simulink model "gap_generation_platoon"  (R2019a)
settings: Solver=VariableStepAuto  StartTime=0.0  StopTime=50  RelTol=1e-3
libraries: simulink x68, powerlib_meascontrol x7, autolibshared x7
(part 3 of 3)

== system gap_generation_platoon/p2/ACC ==
  note: If there's no leader or the leader
      | is too far away, use velocity control
  note: Velocity control
  note: Switch logic (veh foll to vel control)
  note: Vehicle following
  currentStates : Inport
  leaderStates : Inport  Port=2
  lcFlag : Inport  Port=3
  ACC outputs : Scope  NumInputPorts=3
  AND : Logic  IconShape=distinctive  AllPortsSameDT=off  OutDataTypeStr=boolean
  AND1 : Logic  IconShape=distinctive  AllPortsSameDT=off  OutDataTypeStr=boolean
  Anti-windup gain : Gain  Gain=sqrt(Ki/Kd)
  Bus Selector : BusSelector  OutputSignals=X,Xdot,u
  Bus Selector1 : BusSelector  OutputSignals=X,Xdot
  Compare To Constant : simulink/Logic and Bit Operations/Compare To Constant  relop=<  const=2*maxHeadwayError  OutDataTypeStr=boolean
  Compare To Constant1 : simulink/Logic and Bit Operations/Compare To Constant  relop=>  const=0  OutDataTypeStr=boolean
  Gain3 : Gain  Gain=velFilterGain
  Headway error : Subsystem
  Integrator : Integrator  ExternalReset=either
  Integrator1 : Integrator  InitialCondition=vx0
  Integrator2 : Integrator
  Kd : Gain  Gain=Kd
  Ki : Gain  Gain=Ki
  Kp : Gain  Gain=Kp
  Mux : Mux  Inputs=2
  NOT : Logic  Operator=NOT  IconShape=distinctive  AllPortsSameDT=off  OutDataTypeStr=boolean
  Rate Limiter : RateLimiter  RisingSlewLimit=maxJerk  FallingSlewLimit=minJerk  SampleTimeMode=inherited
  Saturation : Saturate  UpperLimit=maxAcceleration  LowerLimit=minAcceleration
  Saturation1 : Saturate  UpperLimit=maxHeadwayError  LowerLimit=minHeadwayError
  Scope : Scope  NumInputPorts=3
  Sum : Sum  Inputs=-+|
  Sum1 : Sum  Inputs=+++
  Sum2 : Sum  Inputs=|+-
  Sum3 : Sum
  Sum4 : Sum  Inputs=+-
  Sum5 : Sum  Inputs=-+|
  Switch : Switch  Criteria=u2 > Threshold
  Switch1 : Switch  Criteria=u2 > Threshold
  comf saturation : Saturate  UpperLimit=maxAcceleration/2  LowerLimit=minAcceleration/4
  safe saturation : Saturate  UpperLimit=maxAcceleration  LowerLimit=minAcceleration
  velKi : Gain  Gain=velKi
  velKp : Gain  Gain=velKp
  u : Outport
  errors : Outport  Port=2
  gap : Outport  Port=3
  wires:
  comf saturation/1 -> Switch1/1
  safe saturation/1 -> Switch1/3
  Switch1/1 -> Rate Limiter/1
  AND1/1 -> Switch1/2
  [lcFlag] -> AND1/2
  NOT/1 -> AND1/1
  [unsafeFlag] -> NOT/1
  Headway error/3(unsafeFlag) -> [unsafeFlag]
  [realInput] -> Sum4/2
  Bus Selector/3 -> [realInput]  "<u>"
  Bus Selector1/1 -> Headway error/3(xl), Compare To Constant1/1  "<X>"
  leaderStates/1 -> Bus Selector1/1
  Bus Selector/1 -> Headway error/1(xf)  "<X>"
  currentStates/1 -> Bus Selector/1
  lcFlag/1 -> Headway error/4(lcFlag), [lcFlag]
  Compare To Constant1/1 -> AND/1
  Compare To Constant/1 -> AND/2
  AND/1 -> ACC outputs/2, Switch/2, Integrator/2
  Anti-windup gain/1 -> Sum5/1
  Integrator/1 -> Scope/1, Sum1/1
  Ki/1 -> Sum5/2
  velKp/1 -> Sum3/1
  Rate Limiter/1 -> u/1  "sat(u)"
  Sum5/1 -> Integrator/1
  Sum4/1 -> Anti-windup gain/1
  Mux/1 -> errors/1
  Sum/1 -> Integrator2/1, velKp/1, Kd/1, Mux/2
  Sum3/1 -> Switch/3, ACC outputs/3
  Sum1/1 -> ACC outputs/1, Switch/1
  Switch/1 -> comf saturation/1, safe saturation/1, Sum4/1  "u"
  velKi/1 -> Sum3/2
  Integrator2/1 -> velKi/1
  Headway error/2("gap ") -> gap/1
  Saturation1/1 -> Ki/1, Kp/1
  Sum2/1 -> Gain3/1
  Bus Selector1/2 -> Sum2/1  "<Xdot>"
  Integrator1/1 -> Sum/2, Sum2/2
  Saturation/1 -> Integrator1/1
  Gain3/1 -> Saturation/1
  Kp/1 -> Sum1/2, Scope/2
  Kd/1 -> Sum1/3, Scope/3
  Bus Selector/2 -> Sum/1, Headway error/2(vf)  "<Xdot>"
  Headway error/1(eh) -> Compare To Constant/1, Mux/1, Saturation1/1

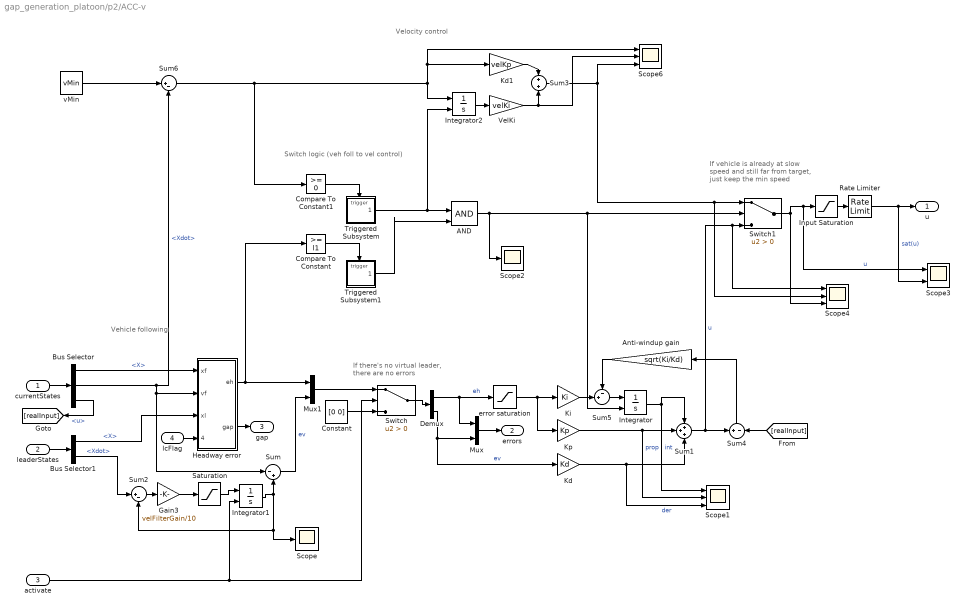
== system gap_generation_platoon/p2/ACC-v ==
  note: If there's no virtual leader,
      | there are no errors
  note: If vehicle is already at slow
      | speed and still far from target,
      | just keep the min speed
  note: Velocity control
  note: Switch logic (veh foll to vel control)
  note: Vehicle following
  currentStates : Inport
  leaderStates : Inport  Port=2
  activate : Inport  Port=3
  lcFlag : Inport  Port=4
  AND : Logic  IconShape=distinctive  AllPortsSameDT=off  OutDataTypeStr=boolean
  Anti-windup gain : Gain  Gain=sqrt(Ki/Kd)
  Bus Selector : BusSelector  OutputSignals=X,Xdot,u
  Bus Selector1 : BusSelector  OutputSignals=X,Xdot
  Compare To Constant : simulink/Logic and Bit Operations/Compare To Constant  relop=>=  const=l1  OutDataTypeStr=boolean
  Compare To Constant1 : simulink/Logic and Bit Operations/Compare To Constant  relop=>=  const=0  OutDataTypeStr=boolean
  Constant : Constant  Value=[0 0]
  Demux : Demux  Outputs=2
  Gain3 : Gain  Gain=velFilterGain/10
  Headway error : Subsystem
  Input Saturation : Saturate  UpperLimit=maxAcceleration/2  LowerLimit=minAcceleration/4
  Integrator : Integrator  ExternalReset=falling
  Integrator1 : Integrator  ExternalReset=rising  InitialCondition=vx0
  Integrator2 : Integrator  ExternalReset=rising
  Kd : Gain  Gain=Kd
  Kd1 : Gain  Gain=velKp
  Ki : Gain  Gain=Ki
  Kp : Gain  Gain=Kp
  Mux : Mux  Inputs=2
  Mux1 : Mux  Inputs=2
  Rate Limiter : RateLimiter  RisingSlewLimit=maxJerk/2  FallingSlewLimit=minJerk/3  SampleTimeMode=inherited
  Saturation : Saturate  UpperLimit=maxAcceleration  LowerLimit=minAcceleration
  Scope : Scope
  Scope1 : Scope  NumInputPorts=3
  Scope2 : Scope
  Scope3 : Scope  NumInputPorts=2
  Scope4 : Scope  NumInputPorts=3
  Scope6 : Scope  NumInputPorts=3
  Sum : Sum  Inputs=|-+
  Sum1 : Sum  Inputs=+++
  Sum2 : Sum  Inputs=|+-
  Sum3 : Sum
  Sum4 : Sum  Inputs=+-
  Sum5 : Sum  Inputs=-+|
  Sum6 : Sum  Inputs=|+-
  Switch : Switch  Criteria=u2 > Threshold
  Switch1 : Switch  Criteria=u2 > Threshold
  Triggered Subsystem : Subsystem  TreatAsAtomicUnit=on
  Triggered Subsystem1 : Subsystem  TreatAsAtomicUnit=on
  VelKi : Gain  Gain=velKi
  error saturation : Saturate  UpperLimit=maxHeadwayError  LowerLimit=minHeadwayError/10
  vMin : Constant  Value=vMin
  u : Outport
  errors : Outport  Port=2
  gap : Outport  Port=3
  wires:
  AND/1 -> Scope2/1, Integrator/2, Switch1/2
  Triggered Subsystem1/1(Out1) -> AND/2
  lcFlag/1 -> Headway error/4(lcFlag)
  Bus Selector/3 -> [realInput]  "<u>"
  Bus Selector1/1 -> Headway error/3(xl)  "<X>"
  leaderStates/1 -> Bus Selector1/1
  Bus Selector/2 -> Sum/1, Headway error/2(vf), Sum6/2  "<Xdot>"
  Bus Selector/1 -> Headway error/1(xf)  "<X>"
  currentStates/1 -> Bus Selector/1
  [realInput] -> Sum4/2
  Triggered Subsystem/1(Out1) -> Integrator2/2, AND/1
  Sum5/1 -> Integrator/1
  error saturation/1 -> Ki/1, Kp/1
  Switch1/1 -> Scope4/3, Input Saturation/1, Scope3/1  "u"
  vMin/1 -> Sum6/1
  VelKi/1 -> Sum3/2, Scope6/2
  Kd1/1 -> Sum3/1
  Integrator2/1 -> VelKi/1
  Sum3/1 -> Switch1/1, Scope4/2, Scope6/3
  Sum6/1 -> Compare To Constant1/1, Integrator2/1, Kd1/1, Scope6/1
  Compare To Constant/1 -> Triggered Subsystem1/Trigger
  Compare To Constant1/1 -> Triggered Subsystem/Trigger
  Rate Limiter/1 -> u/1, Scope3/2  "sat(u)"
  Constant/1 -> Switch/3
  activate/1 -> Integrator1/2, Switch/2
  Mux1/1 -> Switch/1
  Switch/1 -> Demux/1
  Demux/2 -> Kd/1, Mux/2  "ev"
  Anti-windup gain/1 -> Sum5/1
  Ki/1 -> Sum5/2
  Sum4/1 -> Anti-windup gain/1
  Integrator/1 -> Scope1/1, Sum1/1  "int"
  Input Saturation/1 -> Rate Limiter/1
  Mux/1 -> errors/1
  Sum/1 -> Mux1/2  "ev"
  Sum1/1 -> Sum4/1, Switch1/3, Scope4/1  "u"
  Headway error/2("gap ") -> gap/1
  Demux/1 -> Mux/1, error saturation/1  "eh"
  Sum2/1 -> Gain3/1
  Bus Selector1/2 -> Sum2/1  "<Xdot>"
  Integrator1/1 -> Sum/2, Sum2/2, Scope/1
  Saturation/1 -> Integrator1/1
  Gain3/1 -> Saturation/1
  Kp/1 -> Sum1/2, Scope1/2  "prop"
  Kd/1 -> Sum1/3, Scope1/3  "der"
  Headway error/1(eh) -> Compare To Constant/1, Mux1/1

== system gap_generation_platoon/p2/Detect steady state ==
  errors : Inport
  virtual errors : Inport  Port=2
  ACC-v active : Inport  Port=3
  AND1 : Logic  IconShape=distinctive  AllPortsSameDT=off  OutDataTypeStr=boolean
  AND2 : Logic  IconShape=distinctive  AllPortsSameDT=off  OutDataTypeStr=boolean
  AND5 : Logic  IconShape=distinctive  AllPortsSameDT=off  OutDataTypeStr=boolean
  Abs : Abs
  Abs1 : Abs  ZeroCross=off
  Abs2 : Abs
  Abs3 : Abs  ZeroCross=off
  Compare To Constant{,1..3} (4 alike) : simulink/Logic and Bit Operations/Compare To Constant  relop=<=  const=0.5  OutDataTypeStr=boolean
  Demux : Demux  Outputs=2
  OR : Logic  Operator=OR  IconShape=distinctive  AllPortsSameDT=off  OutDataTypeStr=boolean
  Subsystem : Subsystem
  Transport Delay : TransportDelay
  Transport Delay1 : TransportDelay
  Out1 : Outport
  wires:
  ACC-v active/1 -> Subsystem/Enable
  Subsystem/1(Out1) -> OR/2
  virtual errors/1 -> Subsystem/1(virtual errors)
  AND5/1 -> OR/1
  OR/1 -> Out1/1
  AND2/1 -> AND5/2
  AND1/1 -> AND5/1
  Compare To Constant2/1 -> AND2/2
  Compare To Constant3/1 -> AND2/1
  Compare To Constant/1 -> AND1/2
  Compare To Constant1/1 -> AND1/1
  Demux/2 -> Transport Delay1/1, Abs3/1
  Demux/1 -> Transport Delay/1, Abs1/1
  Abs2/1 -> Compare To Constant2/1
  Transport Delay1/1 -> Abs2/1
  Abs3/1 -> Compare To Constant3/1
  errors/1 -> Demux/1
  Abs1/1 -> Compare To Constant1/1
  Transport Delay/1 -> Abs/1
  Abs/1 -> Compare To Constant/1

== system gap_generation_platoon/p2/Triggered Subsystem ==
  In1 : Inport
  Trigger : TriggerPort  VariantControl=Variant
  Out1 : Outport
  wires:
  In1/1 -> Out1/1

== system gap_generation_platoon/p3/ACC ==
  note: Vehicle following
  note: Switch logic (veh foll to vel control)
  note: Velocity control
  note: If there's no leader or the leader
      | is too far away, use velocity control
  currentStates : Inport
  leaderStates : Inport  Port=2
  lcFlag : Inport  Port=3
  ACC outputs : Scope  NumInputPorts=3
  AND : Logic  IconShape=distinctive  AllPortsSameDT=off  OutDataTypeStr=boolean
  AND1 : Logic  IconShape=distinctive  AllPortsSameDT=off  OutDataTypeStr=boolean
  Anti-windup gain : Gain  Gain=sqrt(Ki/Kd)
  Bus Selector : BusSelector  OutputSignals=X,Xdot,u
  Bus Selector1 : BusSelector  OutputSignals=X,Xdot
  Compare To Constant : simulink/Logic and Bit Operations/Compare To Constant  relop=<  const=2*maxHeadwayError  OutDataTypeStr=boolean
  Compare To Constant1 : simulink/Logic and Bit Operations/Compare To Constant  relop=>  const=0  OutDataTypeStr=boolean
  Gain3 : Gain  Gain=velFilterGain
  Headway error : Subsystem
  Integrator : Integrator  ExternalReset=either
  Integrator1 : Integrator  InitialCondition=vx0
  Integrator2 : Integrator
  Kd : Gain  Gain=Kd
  Ki : Gain  Gain=Ki
  Kp : Gain  Gain=Kp
  Mux : Mux  Inputs=2
  NOT : Logic  Operator=NOT  IconShape=distinctive  AllPortsSameDT=off  OutDataTypeStr=boolean
  Rate Limiter : RateLimiter  RisingSlewLimit=maxJerk  FallingSlewLimit=minJerk  SampleTimeMode=inherited
  Saturation : Saturate  UpperLimit=maxAcceleration  LowerLimit=minAcceleration
  Saturation1 : Saturate  UpperLimit=maxHeadwayError  LowerLimit=minHeadwayError
  Scope : Scope  NumInputPorts=3
  Sum : Sum  Inputs=-+|
  Sum1 : Sum  Inputs=+++
  Sum2 : Sum  Inputs=|+-
  Sum3 : Sum
  Sum4 : Sum  Inputs=+-
  Sum5 : Sum  Inputs=-+|
  Switch : Switch  Criteria=u2 > Threshold
  Switch1 : Switch  Criteria=u2 > Threshold
  comf saturation : Saturate  UpperLimit=maxAcceleration/2  LowerLimit=minAcceleration/4
  safe saturation : Saturate  UpperLimit=maxAcceleration  LowerLimit=minAcceleration
  velKi : Gain  Gain=velKi
  velKp : Gain  Gain=velKp
  u : Outport
  errors : Outport  Port=2
  gap : Outport  Port=3
  wires:
  Headway error/1(eh) -> Saturation1/1, Mux/1, Compare To Constant/1
  Bus Selector/2 -> Headway error/2(vf), Sum/1  "<Xdot>"
  Kd/1 -> Scope/3, Sum1/3
  Kp/1 -> Scope/2, Sum1/2
  Gain3/1 -> Saturation/1
  Saturation/1 -> Integrator1/1
  Integrator1/1 -> Sum2/2, Sum/2
  Bus Selector1/2 -> Sum2/1  "<Xdot>"
  Sum2/1 -> Gain3/1
  Saturation1/1 -> Kp/1, Ki/1
  Headway error/2("gap ") -> gap/1
  Integrator2/1 -> velKi/1
  velKi/1 -> Sum3/2
  Switch/1 -> Sum4/1, safe saturation/1, comf saturation/1  "u"
  Sum1/1 -> Switch/1, ACC outputs/1
  Sum3/1 -> ACC outputs/3, Switch/3
  Sum/1 -> Mux/2, Kd/1, velKp/1, Integrator2/1
  Mux/1 -> errors/1
  Sum4/1 -> Anti-windup gain/1
  Sum5/1 -> Integrator/1
  Rate Limiter/1 -> u/1  "sat(u)"
  velKp/1 -> Sum3/1
  Ki/1 -> Sum5/2
  Integrator/1 -> Sum1/1, Scope/1
  Anti-windup gain/1 -> Sum5/1
  AND/1 -> Integrator/2, Switch/2, ACC outputs/2
  Compare To Constant/1 -> AND/2
  Compare To Constant1/1 -> AND/1
  lcFlag/1 -> [lcFlag], Headway error/4(lcFlag)
  currentStates/1 -> Bus Selector/1
  Bus Selector/1 -> Headway error/1(xf)  "<X>"
  leaderStates/1 -> Bus Selector1/1
  Bus Selector1/1 -> Compare To Constant1/1, Headway error/3(xl)  "<X>"
  Bus Selector/3 -> [realInput]  "<u>"
  [realInput] -> Sum4/2
  Headway error/3(unsafeFlag) -> [unsafeFlag]
  [unsafeFlag] -> NOT/1
  NOT/1 -> AND1/1
  [lcFlag] -> AND1/2
  AND1/1 -> Switch1/2
  Switch1/1 -> Rate Limiter/1
  safe saturation/1 -> Switch1/3
  comf saturation/1 -> Switch1/1

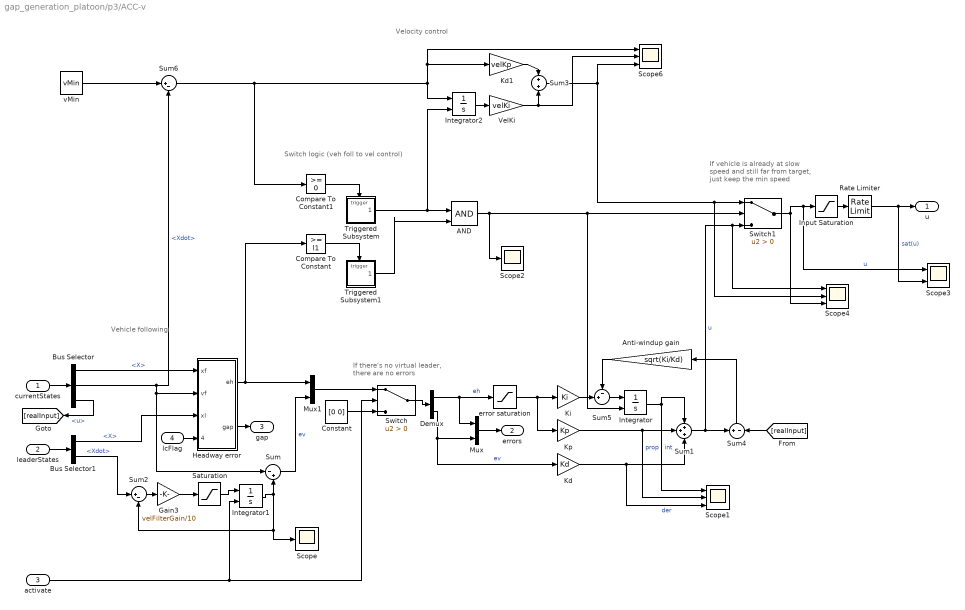
== system gap_generation_platoon/p3/ACC-v ==
  note: Vehicle following
  note: Switch logic (veh foll to vel control)
  note: Velocity control
  note: If vehicle is already at slow
      | speed and still far from target,
      | just keep the min speed
  note: If there's no virtual leader,
      | there are no errors
  currentStates : Inport
  leaderStates : Inport  Port=2
  activate : Inport  Port=3
  lcFlag : Inport  Port=4
  AND : Logic  IconShape=distinctive  AllPortsSameDT=off  OutDataTypeStr=boolean
  Anti-windup gain : Gain  Gain=sqrt(Ki/Kd)
  Bus Selector : BusSelector  OutputSignals=X,Xdot,u
  Bus Selector1 : BusSelector  OutputSignals=X,Xdot
  Compare To Constant : simulink/Logic and Bit Operations/Compare To Constant  relop=>=  const=l1  OutDataTypeStr=boolean
  Compare To Constant1 : simulink/Logic and Bit Operations/Compare To Constant  relop=>=  const=0  OutDataTypeStr=boolean
  Constant : Constant  Value=[0 0]
  Demux : Demux  Outputs=2
  Gain3 : Gain  Gain=velFilterGain/10
  Headway error : Subsystem
  Input Saturation : Saturate  UpperLimit=maxAcceleration/2  LowerLimit=minAcceleration/4
  Integrator : Integrator  ExternalReset=falling
  Integrator1 : Integrator  ExternalReset=rising  InitialCondition=vx0
  Integrator2 : Integrator  ExternalReset=rising
  Kd : Gain  Gain=Kd
  Kd1 : Gain  Gain=velKp
  Ki : Gain  Gain=Ki
  Kp : Gain  Gain=Kp
  Mux : Mux  Inputs=2
  Mux1 : Mux  Inputs=2
  Rate Limiter : RateLimiter  RisingSlewLimit=maxJerk/2  FallingSlewLimit=minJerk/3  SampleTimeMode=inherited
  Saturation : Saturate  UpperLimit=maxAcceleration  LowerLimit=minAcceleration
  Scope : Scope
  Scope1 : Scope  NumInputPorts=3
  Scope2 : Scope
  Scope3 : Scope  NumInputPorts=2
  Scope4 : Scope  NumInputPorts=3
  Scope6 : Scope  NumInputPorts=3
  Sum : Sum  Inputs=|-+
  Sum1 : Sum  Inputs=+++
  Sum2 : Sum  Inputs=|+-
  Sum3 : Sum
  Sum4 : Sum  Inputs=+-
  Sum5 : Sum  Inputs=-+|
  Sum6 : Sum  Inputs=|+-
  Switch : Switch  Criteria=u2 > Threshold
  Switch1 : Switch  Criteria=u2 > Threshold
  Triggered Subsystem : Subsystem  TreatAsAtomicUnit=on
  Triggered Subsystem1 : Subsystem  TreatAsAtomicUnit=on
  VelKi : Gain  Gain=velKi
  error saturation : Saturate  UpperLimit=maxHeadwayError  LowerLimit=minHeadwayError/10
  vMin : Constant  Value=vMin
  u : Outport
  errors : Outport  Port=2
  gap : Outport  Port=3
  wires:
  Headway error/1(eh) -> Mux1/1, Compare To Constant/1
  Kd/1 -> Scope1/3, Sum1/3  "der"
  Kp/1 -> Scope1/2, Sum1/2  "prop"
  Gain3/1 -> Saturation/1
  Saturation/1 -> Integrator1/1
  Integrator1/1 -> Scope/1, Sum2/2, Sum/2
  Bus Selector1/2 -> Sum2/1  "<Xdot>"
  Sum2/1 -> Gain3/1
  Demux/1 -> error saturation/1, Mux/1  "eh"
  Headway error/2("gap ") -> gap/1
  Sum1/1 -> Scope4/1, Switch1/3, Sum4/1  "u"
  Sum/1 -> Mux1/2  "ev"
  Mux/1 -> errors/1
  Input Saturation/1 -> Rate Limiter/1
  Integrator/1 -> Sum1/1, Scope1/1  "int"
  Sum4/1 -> Anti-windup gain/1
  Ki/1 -> Sum5/2
  Anti-windup gain/1 -> Sum5/1
  Demux/2 -> Mux/2, Kd/1  "ev"
  Switch/1 -> Demux/1
  Mux1/1 -> Switch/1
  activate/1 -> Switch/2, Integrator1/2
  Constant/1 -> Switch/3
  Rate Limiter/1 -> Scope3/2, u/1  "sat(u)"
  Compare To Constant1/1 -> Triggered Subsystem/Trigger
  Compare To Constant/1 -> Triggered Subsystem1/Trigger
  Sum6/1 -> Scope6/1, Kd1/1, Integrator2/1, Compare To Constant1/1
  Sum3/1 -> Scope6/3, Scope4/2, Switch1/1
  Integrator2/1 -> VelKi/1
  Kd1/1 -> Sum3/1
  VelKi/1 -> Scope6/2, Sum3/2
  vMin/1 -> Sum6/1
  Switch1/1 -> Scope3/1, Input Saturation/1, Scope4/3  "u"
  error saturation/1 -> Kp/1, Ki/1
  Sum5/1 -> Integrator/1
  Triggered Subsystem/1(Out1) -> AND/1, Integrator2/2
  [realInput] -> Sum4/2
  currentStates/1 -> Bus Selector/1
  Bus Selector/1 -> Headway error/1(xf)  "<X>"
  Bus Selector/2 -> Sum6/2, Headway error/2(vf), Sum/1  "<Xdot>"
  leaderStates/1 -> Bus Selector1/1
  Bus Selector1/1 -> Headway error/3(xl)  "<X>"
  Bus Selector/3 -> [realInput]  "<u>"
  lcFlag/1 -> Headway error/4(lcFlag)
  Triggered Subsystem1/1(Out1) -> AND/2
  AND/1 -> Switch1/2, Integrator/2, Scope2/1

== system gap_generation_platoon/p3/Detect steady state ==
  errors : Inport
  virtual errors : Inport  Port=2
  ACC-v active : Inport  Port=3
  AND1 : Logic  IconShape=distinctive  AllPortsSameDT=off  OutDataTypeStr=boolean
  AND2 : Logic  IconShape=distinctive  AllPortsSameDT=off  OutDataTypeStr=boolean
  AND5 : Logic  IconShape=distinctive  AllPortsSameDT=off  OutDataTypeStr=boolean
  Abs : Abs
  Abs1 : Abs  ZeroCross=off
  Abs2 : Abs
  Abs3 : Abs  ZeroCross=off
  Compare To Constant{,1..3} (4 alike) : simulink/Logic and Bit Operations/Compare To Constant  relop=<=  const=0.5  OutDataTypeStr=boolean
  Demux : Demux  Outputs=2
  OR : Logic  Operator=OR  IconShape=distinctive  AllPortsSameDT=off  OutDataTypeStr=boolean
  Subsystem : Subsystem
  Transport Delay : TransportDelay
  Transport Delay1 : TransportDelay
  Out1 : Outport
  wires:
  Abs/1 -> Compare To Constant/1
  Transport Delay/1 -> Abs/1
  Abs1/1 -> Compare To Constant1/1
  errors/1 -> Demux/1
  Abs3/1 -> Compare To Constant3/1
  Transport Delay1/1 -> Abs2/1
  Abs2/1 -> Compare To Constant2/1
  Demux/1 -> Abs1/1, Transport Delay/1
  Demux/2 -> Abs3/1, Transport Delay1/1
  Compare To Constant1/1 -> AND1/1
  Compare To Constant/1 -> AND1/2
  Compare To Constant3/1 -> AND2/1
  Compare To Constant2/1 -> AND2/2
  AND1/1 -> AND5/1
  AND2/1 -> AND5/2
  OR/1 -> Out1/1
  AND5/1 -> OR/1
  virtual errors/1 -> Subsystem/1(virtual errors)
  Subsystem/1(Out1) -> OR/2
  ACC-v active/1 -> Subsystem/Enable

== system gap_generation_platoon/p3/Triggered Subsystem ==
  In1 : Inport
  Trigger : TriggerPort  VariantControl=Variant
  Out1 : Outport
  wires:
  In1/1 -> Out1/1

== system gap_generation_platoon/Fd/ACC/Headway error ==
  xf : Inport
  vf : Inport  Port=2
  xl : Inport  Port=3
  lcFlag : Inport  Port=4
  Compare To Constant : simulink/Logic and Bit Operations/Compare To Constant  relop=<=  const=0  OutDataTypeStr=boolean
  Demux : Demux  Outputs=2
  Demux1 : Demux  Outputs=2
  Integrator : Integrator  InitialCondition=[h d0]
  Multiply : Product
  Mux : Mux  Inputs=2
  Mux1 : Mux  Inputs=2
  Product : Product
  Sum : Sum  Inputs=-+|
  Sum1 : Sum  Inputs=++|
  Sum2 : Sum  Inputs=+-|
  Sum3 : Sum  Inputs=|++
  Sum4 : Sum  Inputs=|+-
  Sum5 : Sum  Inputs=+-|
  Sum6 : Sum  Inputs=|++
  Switch : Switch  Criteria=u2 > Threshold
  d0 : Constant  Value=d0
  d0Lc : Constant  Value=d0Lc
  h : Constant  Value=h
  hFilterGain : Gain  Gain=hFilterGain
  hLc : Constant  Value=hLc
  vLen : Constant  Value=lr+lf
  eh : Outport
  "gap " : Outport  Port=2
  unsafeFlag : Outport  Port=3
  wires:
  vLen/1 -> Sum1/1
  Multiply/1 -> Sum3/1
  Sum/1 -> Sum5/1, "gap "/1, Sum2/1  "gap"
  xf/1 -> Sum1/2
  Sum3/1 -> Sum2/2  "desired  gap"
  vf/1 -> Product/1, Multiply/1
  Sum1/1 -> Sum/1  "x (front bumber)"
  xl/1 -> Sum/2
  h/1 -> Mux/1
  Switch/1 -> Sum4/1
  Sum4/1 -> hFilterGain/1
  Integrator/1 -> Sum4/2, Demux/1
  lcFlag/1 -> Switch/2
  Sum2/1 -> eh/1
  d0/1 -> Mux/2
  Mux/1 -> Demux1/1, Switch/3  "min safe gap"
  hLc/1 -> Mux1/1
  d0Lc/1 -> Mux1/2
  Mux1/1 -> Switch/1
  Demux/1 -> Multiply/2  "time headway"
  Demux/2 -> Sum3/2  "gap at  standstill"
  hFilterGain/1 -> Integrator/1
  Sum5/1 -> Compare To Constant/1
  Compare To Constant/1 -> unsafeFlag/1
  Demux1/1 -> Product/2  "time headway"
  Product/1 -> Sum6/1
  Demux1/2 -> Sum6/2  "gap at  standstill"
  Sum6/1 -> Sum5/2  "safe  gap"

== system gap_generation_platoon/Fd/ACC-v/Headway error ==
  xf : Inport
  vf : Inport  Port=2
  xl : Inport  Port=3
  lcFlag : Inport  Port=4
  Demux : Demux  Outputs=2
  Integrator : Integrator  InitialCondition=h
  Multiply : Product
  Mux : Mux  Inputs=2
  Mux1 : Mux  Inputs=2
  Sum : Sum  Inputs=-+|
  Sum1 : Sum  Inputs=++|
  Sum2 : Sum  Inputs=+-|
  Sum3 : Sum  Inputs=|++
  Sum4 : Sum  Inputs=|+-
  Switch : Switch  Criteria=u2 > Threshold
  d0 : Constant  Value=d0
  d0Lc : Constant  Value=d0Lc
  h : Constant  Value=h
  hFilterGain : Gain  Gain=hFilterGain
  hLc : Constant  Value=hLc
  vLen : Constant  Value=lr+lf
  eh : Outport
  "gap " : Outport  Port=2
  wires:
  vLen/1 -> Sum1/1
  Multiply/1 -> Sum3/1
  Sum/1 -> "gap "/1, Sum2/1  "gap"
  xf/1 -> Sum1/2
  Sum3/1 -> Sum2/2  "desired  gap"
  vf/1 -> Multiply/1
  Sum1/1 -> Sum/1  "x (front bumber)"
  xl/1 -> Sum/2
  h/1 -> Mux/1
  Switch/1 -> Sum4/1
  hFilterGain/1 -> Integrator/1
  Sum4/1 -> hFilterGain/1
  Integrator/1 -> Sum4/2, Demux/1
  lcFlag/1 -> Switch/2
  Sum2/1 -> eh/1
  d0/1 -> Mux/2
  Mux/1 -> Switch/3
  hLc/1 -> Mux1/1
  d0Lc/1 -> Mux1/2
  Mux1/1 -> Switch/1
  Demux/1 -> Multiply/2  "time headway"
  Demux/2 -> Sum3/2  "gap at  standstill"

== system gap_generation_platoon/Fd/ACC-v/Triggered Subsystem ==
  Trigger : TriggerPort  VariantControl=Variant
  Constant : Constant
  Out1 : Outport  InitialOutput=0
  wires:
  Constant/1 -> Out1/1

== system gap_generation_platoon/Fd/ACC-v/Triggered Subsystem1 ==
  Trigger : TriggerPort  VariantControl=Variant
  Constant : Constant  Value=0
  Out1 : Outport  InitialOutput=1
  wires:
  Constant/1 -> Out1/1

== system gap_generation_platoon/Fo/ACC/Headway error ==
  xf : Inport
  vf : Inport  Port=2
  xl : Inport  Port=3
  lcFlag : Inport  Port=4
  Compare To Constant : simulink/Logic and Bit Operations/Compare To Constant  relop=<=  const=0  OutDataTypeStr=boolean
  Demux : Demux  Outputs=2
  Demux1 : Demux  Outputs=2
  Integrator : Integrator  InitialCondition=[h d0]
  Multiply : Product
  Mux : Mux  Inputs=2
  Mux1 : Mux  Inputs=2
  Product : Product
  Sum : Sum  Inputs=-+|
  Sum1 : Sum  Inputs=++|
  Sum2 : Sum  Inputs=+-|
  Sum3 : Sum  Inputs=|++
  Sum4 : Sum  Inputs=|+-
  Sum5 : Sum  Inputs=+-|
  Sum6 : Sum  Inputs=|++
  Switch : Switch  Criteria=u2 > Threshold
  d0 : Constant  Value=d0
  d0Lc : Constant  Value=d0Lc
  h : Constant  Value=h
  hFilterGain : Gain  Gain=hFilterGain
  hLc : Constant  Value=hLc
  vLen : Constant  Value=lr+lf
  eh : Outport
  "gap " : Outport  Port=2
  unsafeFlag : Outport  Port=3
  wires:
  Sum6/1 -> Sum5/2  "safe  gap"
  Demux1/2 -> Sum6/2  "gap at  standstill"
  Product/1 -> Sum6/1
  Demux1/1 -> Product/2  "time headway"
  Compare To Constant/1 -> unsafeFlag/1
  Sum5/1 -> Compare To Constant/1
  hFilterGain/1 -> Integrator/1
  Demux/2 -> Sum3/2  "gap at  standstill"
  Demux/1 -> Multiply/2  "time headway"
  Mux1/1 -> Switch/1
  d0Lc/1 -> Mux1/2
  hLc/1 -> Mux1/1
  Mux/1 -> Switch/3, Demux1/1  "min safe gap"
  d0/1 -> Mux/2
  Sum2/1 -> eh/1
  lcFlag/1 -> Switch/2
  Integrator/1 -> Demux/1, Sum4/2
  Sum4/1 -> hFilterGain/1
  Switch/1 -> Sum4/1
  h/1 -> Mux/1
  xl/1 -> Sum/2
  Sum1/1 -> Sum/1  "x (front bumber)"
  vf/1 -> Multiply/1, Product/1
  Sum3/1 -> Sum2/2  "desired  gap"
  xf/1 -> Sum1/2
  Sum/1 -> Sum2/1, "gap "/1, Sum5/1  "gap"
  Multiply/1 -> Sum3/1
  vLen/1 -> Sum1/1

== system gap_generation_platoon/Fo/ACC-v/Headway error ==
  xf : Inport
  vf : Inport  Port=2
  xl : Inport  Port=3
  lcFlag : Inport  Port=4
  Demux : Demux  Outputs=2
  Integrator : Integrator  InitialCondition=h
  Multiply : Product
  Mux : Mux  Inputs=2
  Mux1 : Mux  Inputs=2
  Sum : Sum  Inputs=-+|
  Sum1 : Sum  Inputs=++|
  Sum2 : Sum  Inputs=+-|
  Sum3 : Sum  Inputs=|++
  Sum4 : Sum  Inputs=|+-
  Switch : Switch  Criteria=u2 > Threshold
  d0 : Constant  Value=d0
  d0Lc : Constant  Value=d0Lc
  h : Constant  Value=h
  hFilterGain : Gain  Gain=hFilterGain
  hLc : Constant  Value=hLc
  vLen : Constant  Value=lr+lf
  eh : Outport
  "gap " : Outport  Port=2
  wires:
  Demux/2 -> Sum3/2  "gap at  standstill"
  Demux/1 -> Multiply/2  "time headway"
  Mux1/1 -> Switch/1
  d0Lc/1 -> Mux1/2
  hLc/1 -> Mux1/1
  Mux/1 -> Switch/3
  d0/1 -> Mux/2
  Sum2/1 -> eh/1
  lcFlag/1 -> Switch/2
  Integrator/1 -> Demux/1, Sum4/2
  Sum4/1 -> hFilterGain/1
  hFilterGain/1 -> Integrator/1
  Switch/1 -> Sum4/1
  h/1 -> Mux/1
  xl/1 -> Sum/2
  Sum1/1 -> Sum/1  "x (front bumber)"
  vf/1 -> Multiply/1
  Sum3/1 -> Sum2/2  "desired  gap"
  xf/1 -> Sum1/2
  Sum/1 -> Sum2/1, "gap "/1  "gap"
  Multiply/1 -> Sum3/1
  vLen/1 -> Sum1/1

== system gap_generation_platoon/Fo/ACC-v/Triggered Subsystem ==
  Trigger : TriggerPort  VariantControl=Variant
  Constant : Constant
  Out1 : Outport  InitialOutput=0
  wires:
  Constant/1 -> Out1/1

== system gap_generation_platoon/Fo/ACC-v/Triggered Subsystem1 ==
  Trigger : TriggerPort  VariantControl=Variant
  Constant : Constant  Value=0
  Out1 : Outport  InitialOutput=1
  wires:
  Constant/1 -> Out1/1

== system gap_generation_platoon/Ld/ACC/Headway error ==
  xf : Inport
  vf : Inport  Port=2
  xl : Inport  Port=3
  lcFlag : Inport  Port=4
  Compare To Constant : simulink/Logic and Bit Operations/Compare To Constant  relop=<=  const=0  OutDataTypeStr=boolean
  Demux : Demux  Outputs=2
  Demux1 : Demux  Outputs=2
  Integrator : Integrator  InitialCondition=[h d0]
  Multiply : Product
  Mux : Mux  Inputs=2
  Mux1 : Mux  Inputs=2
  Product : Product
  Sum : Sum  Inputs=-+|
  Sum1 : Sum  Inputs=++|
  Sum2 : Sum  Inputs=+-|
  Sum3 : Sum  Inputs=|++
  Sum4 : Sum  Inputs=|+-
  Sum5 : Sum  Inputs=+-|
  Sum6 : Sum  Inputs=|++
  Switch : Switch  Criteria=u2 > Threshold
  d0 : Constant  Value=d0
  d0Lc : Constant  Value=d0Lc
  h : Constant  Value=h
  hFilterGain : Gain  Gain=hFilterGain
  hLc : Constant  Value=hLc
  vLen : Constant  Value=lr+lf
  eh : Outport
  "gap " : Outport  Port=2
  unsafeFlag : Outport  Port=3
  wires:
  Sum6/1 -> Sum5/2  "safe  gap"
  Demux1/2 -> Sum6/2  "gap at  standstill"
  Product/1 -> Sum6/1
  Demux1/1 -> Product/2  "time headway"
  Compare To Constant/1 -> unsafeFlag/1
  Sum5/1 -> Compare To Constant/1
  hFilterGain/1 -> Integrator/1
  Demux/2 -> Sum3/2  "gap at  standstill"
  Demux/1 -> Multiply/2  "time headway"
  Mux1/1 -> Switch/1
  d0Lc/1 -> Mux1/2
  hLc/1 -> Mux1/1
  Mux/1 -> Switch/3, Demux1/1  "min safe gap"
  d0/1 -> Mux/2
  Sum2/1 -> eh/1
  lcFlag/1 -> Switch/2
  Integrator/1 -> Demux/1, Sum4/2
  Sum4/1 -> hFilterGain/1
  Switch/1 -> Sum4/1
  h/1 -> Mux/1
  xl/1 -> Sum/2
  Sum1/1 -> Sum/1  "x (front bumber)"
  vf/1 -> Multiply/1, Product/1
  Sum3/1 -> Sum2/2  "desired  gap"
  xf/1 -> Sum1/2
  Sum/1 -> Sum2/1, "gap "/1, Sum5/1  "gap"
  Multiply/1 -> Sum3/1
  vLen/1 -> Sum1/1

== system gap_generation_platoon/Ld/ACC-v/Headway error ==
  xf : Inport
  vf : Inport  Port=2
  xl : Inport  Port=3
  lcFlag : Inport  Port=4
  Demux : Demux  Outputs=2
  Integrator : Integrator  InitialCondition=h
  Multiply : Product
  Mux : Mux  Inputs=2
  Mux1 : Mux  Inputs=2
  Sum : Sum  Inputs=-+|
  Sum1 : Sum  Inputs=++|
  Sum2 : Sum  Inputs=+-|
  Sum3 : Sum  Inputs=|++
  Sum4 : Sum  Inputs=|+-
  Switch : Switch  Criteria=u2 > Threshold
  d0 : Constant  Value=d0
  d0Lc : Constant  Value=d0Lc
  h : Constant  Value=h
  hFilterGain : Gain  Gain=hFilterGain
  hLc : Constant  Value=hLc
  vLen : Constant  Value=lr+lf
  eh : Outport
  "gap " : Outport  Port=2
  wires:
  Demux/2 -> Sum3/2  "gap at  standstill"
  Demux/1 -> Multiply/2  "time headway"
  Mux1/1 -> Switch/1
  d0Lc/1 -> Mux1/2
  hLc/1 -> Mux1/1
  Mux/1 -> Switch/3
  d0/1 -> Mux/2
  Sum2/1 -> eh/1
  lcFlag/1 -> Switch/2
  Integrator/1 -> Demux/1, Sum4/2
  Sum4/1 -> hFilterGain/1
  hFilterGain/1 -> Integrator/1
  Switch/1 -> Sum4/1
  h/1 -> Mux/1
  xl/1 -> Sum/2
  Sum1/1 -> Sum/1  "x (front bumber)"
  vf/1 -> Multiply/1
  Sum3/1 -> Sum2/2  "desired  gap"
  xf/1 -> Sum1/2
  Sum/1 -> Sum2/1, "gap "/1  "gap"
  Multiply/1 -> Sum3/1
  vLen/1 -> Sum1/1

== system gap_generation_platoon/Ld/ACC-v/Triggered Subsystem ==
  Trigger : TriggerPort  VariantControl=Variant
  Constant : Constant
  Out1 : Outport  InitialOutput=0
  wires:
  Constant/1 -> Out1/1

== system gap_generation_platoon/Ld/ACC-v/Triggered Subsystem1 ==
  Trigger : TriggerPort  VariantControl=Variant
  Constant : Constant  Value=0
  Out1 : Outport  InitialOutput=1
  wires:
  Constant/1 -> Out1/1

== system gap_generation_platoon/Lo/ACC/Headway error ==
  xf : Inport
  vf : Inport  Port=2
  xl : Inport  Port=3
  lcFlag : Inport  Port=4
  Compare To Constant : simulink/Logic and Bit Operations/Compare To Constant  relop=<=  const=0  OutDataTypeStr=boolean
  Demux : Demux  Outputs=2
  Demux1 : Demux  Outputs=2
  Integrator : Integrator  InitialCondition=[h d0]
  Multiply : Product
  Mux : Mux  Inputs=2
  Mux1 : Mux  Inputs=2
  Product : Product
  Sum : Sum  Inputs=-+|
  Sum1 : Sum  Inputs=++|
  Sum2 : Sum  Inputs=+-|
  Sum3 : Sum  Inputs=|++
  Sum4 : Sum  Inputs=|+-
  Sum5 : Sum  Inputs=+-|
  Sum6 : Sum  Inputs=|++
  Switch : Switch  Criteria=u2 > Threshold
  d0 : Constant  Value=d0
  d0Lc : Constant  Value=d0Lc
  h : Constant  Value=h
  hFilterGain : Gain  Gain=hFilterGain
  hLc : Constant  Value=hLc
  vLen : Constant  Value=lr+lf
  eh : Outport
  "gap " : Outport  Port=2
  unsafeFlag : Outport  Port=3
  wires:
  vLen/1 -> Sum1/1
  Multiply/1 -> Sum3/1
  Sum/1 -> Sum5/1, "gap "/1, Sum2/1  "gap"
  xf/1 -> Sum1/2
  Sum3/1 -> Sum2/2  "desired  gap"
  vf/1 -> Product/1, Multiply/1
  Sum1/1 -> Sum/1  "x (front bumber)"
  xl/1 -> Sum/2
  h/1 -> Mux/1
  Switch/1 -> Sum4/1
  Sum4/1 -> hFilterGain/1
  Integrator/1 -> Sum4/2, Demux/1
  lcFlag/1 -> Switch/2
  Sum2/1 -> eh/1
  d0/1 -> Mux/2
  Mux/1 -> Demux1/1, Switch/3  "min safe gap"
  hLc/1 -> Mux1/1
  d0Lc/1 -> Mux1/2
  Mux1/1 -> Switch/1
  Demux/1 -> Multiply/2  "time headway"
  Demux/2 -> Sum3/2  "gap at  standstill"
  hFilterGain/1 -> Integrator/1
  Sum5/1 -> Compare To Constant/1
  Compare To Constant/1 -> unsafeFlag/1
  Demux1/1 -> Product/2  "time headway"
  Product/1 -> Sum6/1
  Demux1/2 -> Sum6/2  "gap at  standstill"
  Sum6/1 -> Sum5/2  "safe  gap"

== system gap_generation_platoon/Lo/ACC-v/Headway error ==
  xf : Inport
  vf : Inport  Port=2
  xl : Inport  Port=3
  lcFlag : Inport  Port=4
  Demux : Demux  Outputs=2
  Integrator : Integrator  InitialCondition=h
  Multiply : Product
  Mux : Mux  Inputs=2
  Mux1 : Mux  Inputs=2
  Sum : Sum  Inputs=-+|
  Sum1 : Sum  Inputs=++|
  Sum2 : Sum  Inputs=+-|
  Sum3 : Sum  Inputs=|++
  Sum4 : Sum  Inputs=|+-
  Switch : Switch  Criteria=u2 > Threshold
  d0 : Constant  Value=d0
  d0Lc : Constant  Value=d0Lc
  h : Constant  Value=h
  hFilterGain : Gain  Gain=hFilterGain
  hLc : Constant  Value=hLc
  vLen : Constant  Value=lr+lf
  eh : Outport
  "gap " : Outport  Port=2
  wires:
  vLen/1 -> Sum1/1
  Multiply/1 -> Sum3/1
  Sum/1 -> "gap "/1, Sum2/1  "gap"
  xf/1 -> Sum1/2
  Sum3/1 -> Sum2/2  "desired  gap"
  vf/1 -> Multiply/1
  Sum1/1 -> Sum/1  "x (front bumber)"
  xl/1 -> Sum/2
  h/1 -> Mux/1
  Switch/1 -> Sum4/1
  hFilterGain/1 -> Integrator/1
  Sum4/1 -> hFilterGain/1
  Integrator/1 -> Sum4/2, Demux/1
  lcFlag/1 -> Switch/2
  Sum2/1 -> eh/1
  d0/1 -> Mux/2
  Mux/1 -> Switch/3
  hLc/1 -> Mux1/1
  d0Lc/1 -> Mux1/2
  Mux1/1 -> Switch/1
  Demux/1 -> Multiply/2  "time headway"
  Demux/2 -> Sum3/2  "gap at  standstill"

== system gap_generation_platoon/Lo/ACC-v/Triggered Subsystem ==
  Trigger : TriggerPort  VariantControl=Variant
  Constant : Constant
  Out1 : Outport  InitialOutput=0
  wires:
  Constant/1 -> Out1/1

== system gap_generation_platoon/Lo/ACC-v/Triggered Subsystem1 ==
  Trigger : TriggerPort  VariantControl=Variant
  Constant : Constant  Value=0
  Out1 : Outport  InitialOutput=1
  wires:
  Constant/1 -> Out1/1

== system gap_generation_platoon/p1/ACC/Headway error ==
  xf : Inport
  vf : Inport  Port=2
  xl : Inport  Port=3
  lcFlag : Inport  Port=4
  Compare To Constant : simulink/Logic and Bit Operations/Compare To Constant  relop=<=  const=0  OutDataTypeStr=boolean
  Demux : Demux  Outputs=2
  Demux1 : Demux  Outputs=2
  Integrator : Integrator  InitialCondition=[h d0]
  Multiply : Product
  Mux : Mux  Inputs=2
  Mux1 : Mux  Inputs=2
  Product : Product
  Sum : Sum  Inputs=-+|
  Sum1 : Sum  Inputs=++|
  Sum2 : Sum  Inputs=+-|
  Sum3 : Sum  Inputs=|++
  Sum4 : Sum  Inputs=|+-
  Sum5 : Sum  Inputs=+-|
  Sum6 : Sum  Inputs=|++
  Switch : Switch  Criteria=u2 > Threshold
  d0 : Constant  Value=d0
  d0Lc : Constant  Value=d0Lc
  h : Constant  Value=h
  hFilterGain : Gain  Gain=hFilterGain
  hLc : Constant  Value=hLc
  vLen : Constant  Value=lr+lf
  eh : Outport
  "gap " : Outport  Port=2
  unsafeFlag : Outport  Port=3
  wires:
  vLen/1 -> Sum1/1
  Multiply/1 -> Sum3/1
  Sum/1 -> Sum5/1, "gap "/1, Sum2/1  "gap"
  xf/1 -> Sum1/2
  Sum3/1 -> Sum2/2  "desired  gap"
  vf/1 -> Product/1, Multiply/1
  Sum1/1 -> Sum/1  "x (front bumber)"
  xl/1 -> Sum/2
  h/1 -> Mux/1
  Switch/1 -> Sum4/1
  Sum4/1 -> hFilterGain/1
  Integrator/1 -> Sum4/2, Demux/1
  lcFlag/1 -> Switch/2
  Sum2/1 -> eh/1
  d0/1 -> Mux/2
  Mux/1 -> Demux1/1, Switch/3  "min safe gap"
  hLc/1 -> Mux1/1
  d0Lc/1 -> Mux1/2
  Mux1/1 -> Switch/1
  Demux/1 -> Multiply/2  "time headway"
  Demux/2 -> Sum3/2  "gap at  standstill"
  hFilterGain/1 -> Integrator/1
  Sum5/1 -> Compare To Constant/1
  Compare To Constant/1 -> unsafeFlag/1
  Demux1/1 -> Product/2  "time headway"
  Product/1 -> Sum6/1
  Demux1/2 -> Sum6/2  "gap at  standstill"
  Sum6/1 -> Sum5/2  "safe  gap"

== system gap_generation_platoon/p1/ACC-v/Headway error ==
  xf : Inport
  vf : Inport  Port=2
  xl : Inport  Port=3
  lcFlag : Inport  Port=4
  Demux : Demux  Outputs=2
  Integrator : Integrator  InitialCondition=h
  Multiply : Product
  Mux : Mux  Inputs=2
  Mux1 : Mux  Inputs=2
  Sum : Sum  Inputs=-+|
  Sum1 : Sum  Inputs=++|
  Sum2 : Sum  Inputs=+-|
  Sum3 : Sum  Inputs=|++
  Sum4 : Sum  Inputs=|+-
  Switch : Switch  Criteria=u2 > Threshold
  d0 : Constant  Value=d0
  d0Lc : Constant  Value=d0Lc
  h : Constant  Value=h
  hFilterGain : Gain  Gain=hFilterGain
  hLc : Constant  Value=hLc
  vLen : Constant  Value=lr+lf
  eh : Outport
  "gap " : Outport  Port=2
  wires:
  vLen/1 -> Sum1/1
  Multiply/1 -> Sum3/1
  Sum/1 -> "gap "/1, Sum2/1  "gap"
  xf/1 -> Sum1/2
  Sum3/1 -> Sum2/2  "desired  gap"
  vf/1 -> Multiply/1
  Sum1/1 -> Sum/1  "x (front bumber)"
  xl/1 -> Sum/2
  h/1 -> Mux/1
  Switch/1 -> Sum4/1
  hFilterGain/1 -> Integrator/1
  Sum4/1 -> hFilterGain/1
  Integrator/1 -> Sum4/2, Demux/1
  lcFlag/1 -> Switch/2
  Sum2/1 -> eh/1
  d0/1 -> Mux/2
  Mux/1 -> Switch/3
  hLc/1 -> Mux1/1
  d0Lc/1 -> Mux1/2
  Mux1/1 -> Switch/1
  Demux/1 -> Multiply/2  "time headway"
  Demux/2 -> Sum3/2  "gap at  standstill"

== system gap_generation_platoon/p1/ACC-v/Triggered Subsystem ==
  Trigger : TriggerPort  VariantControl=Variant
  Constant : Constant
  Out1 : Outport  InitialOutput=0
  wires:
  Constant/1 -> Out1/1

== system gap_generation_platoon/p1/ACC-v/Triggered Subsystem1 ==
  Trigger : TriggerPort  VariantControl=Variant
  Constant : Constant  Value=0
  Out1 : Outport  InitialOutput=1
  wires:
  Constant/1 -> Out1/1

== system gap_generation_platoon/p1/Detect steady state/Subsystem ==
  virtual errors : Inport
  Enable : EnablePort
  AND3 : Logic  IconShape=distinctive  AllPortsSameDT=off  OutDataTypeStr=boolean
  AND4 : Logic  IconShape=distinctive  AllPortsSameDT=off  OutDataTypeStr=boolean
  AND6 : Logic  IconShape=distinctive  AllPortsSameDT=off  OutDataTypeStr=boolean
  Abs4 : Abs
  Abs5 : Abs  ZeroCross=off
  Abs6 : Abs
  Abs7 : Abs  ZeroCross=off
  Compare To Constant{4..7} (4 alike) : simulink/Logic and Bit Operations/Compare To Constant  relop=<=  const=0.5  OutDataTypeStr=boolean
  Demux1 : Demux  Outputs=2
  Transport Delay2 : TransportDelay
  Transport Delay3 : TransportDelay
  Out1 : Outport  OutputWhenDisabled=reset  InitialOutput=0
  wires:
  Abs7/1 -> Compare To Constant7/1
  Transport Delay3/1 -> Abs6/1
  Demux1/1 -> Transport Delay2/1, Abs5/1
  Compare To Constant6/1 -> AND4/2
  Compare To Constant4/1 -> AND3/2
  Compare To Constant7/1 -> AND4/1
  virtual errors/1 -> Demux1/1
  Demux1/2 -> Abs7/1, Transport Delay3/1
  AND6/1 -> Out1/1
  Abs6/1 -> Compare To Constant6/1
  Compare To Constant5/1 -> AND3/1
  Transport Delay2/1 -> Abs4/1
  Abs5/1 -> Compare To Constant5/1
  AND3/1 -> AND6/1
  Abs4/1 -> Compare To Constant4/1
  AND4/1 -> AND6/2

== system gap_generation_platoon/p2/ACC/Headway error ==
  xf : Inport
  vf : Inport  Port=2
  xl : Inport  Port=3
  lcFlag : Inport  Port=4
  Compare To Constant : simulink/Logic and Bit Operations/Compare To Constant  relop=<=  const=0  OutDataTypeStr=boolean
  Demux : Demux  Outputs=2
  Demux1 : Demux  Outputs=2
  Integrator : Integrator  InitialCondition=[h d0]
  Multiply : Product
  Mux : Mux  Inputs=2
  Mux1 : Mux  Inputs=2
  Product : Product
  Sum : Sum  Inputs=-+|
  Sum1 : Sum  Inputs=++|
  Sum2 : Sum  Inputs=+-|
  Sum3 : Sum  Inputs=|++
  Sum4 : Sum  Inputs=|+-
  Sum5 : Sum  Inputs=+-|
  Sum6 : Sum  Inputs=|++
  Switch : Switch  Criteria=u2 > Threshold
  d0 : Constant  Value=d0
  d0Lc : Constant  Value=d0Lc
  h : Constant  Value=h
  hFilterGain : Gain  Gain=hFilterGain
  hLc : Constant  Value=hLc
  vLen : Constant  Value=lr+lf
  eh : Outport
  "gap " : Outport  Port=2
  unsafeFlag : Outport  Port=3
  wires:
  Sum6/1 -> Sum5/2  "safe  gap"
  Demux1/2 -> Sum6/2  "gap at  standstill"
  Product/1 -> Sum6/1
  Demux1/1 -> Product/2  "time headway"
  Compare To Constant/1 -> unsafeFlag/1
  Sum5/1 -> Compare To Constant/1
  hFilterGain/1 -> Integrator/1
  Demux/2 -> Sum3/2  "gap at  standstill"
  Demux/1 -> Multiply/2  "time headway"
  Mux1/1 -> Switch/1
  d0Lc/1 -> Mux1/2
  hLc/1 -> Mux1/1
  Mux/1 -> Switch/3, Demux1/1  "min safe gap"
  d0/1 -> Mux/2
  Sum2/1 -> eh/1
  lcFlag/1 -> Switch/2
  Integrator/1 -> Demux/1, Sum4/2
  Sum4/1 -> hFilterGain/1
  Switch/1 -> Sum4/1
  h/1 -> Mux/1
  xl/1 -> Sum/2
  Sum1/1 -> Sum/1  "x (front bumber)"
  vf/1 -> Multiply/1, Product/1
  Sum3/1 -> Sum2/2  "desired  gap"
  xf/1 -> Sum1/2
  Sum/1 -> Sum2/1, "gap "/1, Sum5/1  "gap"
  Multiply/1 -> Sum3/1
  vLen/1 -> Sum1/1

== system gap_generation_platoon/p2/ACC-v/Headway error ==
  xf : Inport
  vf : Inport  Port=2
  xl : Inport  Port=3
  lcFlag : Inport  Port=4
  Demux : Demux  Outputs=2
  Integrator : Integrator  InitialCondition=h
  Multiply : Product
  Mux : Mux  Inputs=2
  Mux1 : Mux  Inputs=2
  Sum : Sum  Inputs=-+|
  Sum1 : Sum  Inputs=++|
  Sum2 : Sum  Inputs=+-|
  Sum3 : Sum  Inputs=|++
  Sum4 : Sum  Inputs=|+-
  Switch : Switch  Criteria=u2 > Threshold
  d0 : Constant  Value=d0
  d0Lc : Constant  Value=d0Lc
  h : Constant  Value=h
  hFilterGain : Gain  Gain=hFilterGain
  hLc : Constant  Value=hLc
  vLen : Constant  Value=lr+lf
  eh : Outport
  "gap " : Outport  Port=2
  wires:
  Demux/2 -> Sum3/2  "gap at  standstill"
  Demux/1 -> Multiply/2  "time headway"
  Mux1/1 -> Switch/1
  d0Lc/1 -> Mux1/2
  hLc/1 -> Mux1/1
  Mux/1 -> Switch/3
  d0/1 -> Mux/2
  Sum2/1 -> eh/1
  lcFlag/1 -> Switch/2
  Integrator/1 -> Demux/1, Sum4/2
  Sum4/1 -> hFilterGain/1
  hFilterGain/1 -> Integrator/1
  Switch/1 -> Sum4/1
  h/1 -> Mux/1
  xl/1 -> Sum/2
  Sum1/1 -> Sum/1  "x (front bumber)"
  vf/1 -> Multiply/1
  Sum3/1 -> Sum2/2  "desired  gap"
  xf/1 -> Sum1/2
  Sum/1 -> Sum2/1, "gap "/1  "gap"
  Multiply/1 -> Sum3/1
  vLen/1 -> Sum1/1

== system gap_generation_platoon/p2/ACC-v/Triggered Subsystem ==
  Trigger : TriggerPort  VariantControl=Variant
  Constant : Constant
  Out1 : Outport  InitialOutput=0
  wires:
  Constant/1 -> Out1/1

== system gap_generation_platoon/p2/ACC-v/Triggered Subsystem1 ==
  Trigger : TriggerPort  VariantControl=Variant
  Constant : Constant  Value=0
  Out1 : Outport  InitialOutput=1
  wires:
  Constant/1 -> Out1/1

== system gap_generation_platoon/p2/Detect steady state/Subsystem ==
  virtual errors : Inport
  Enable : EnablePort
  AND3 : Logic  IconShape=distinctive  AllPortsSameDT=off  OutDataTypeStr=boolean
  AND4 : Logic  IconShape=distinctive  AllPortsSameDT=off  OutDataTypeStr=boolean
  AND6 : Logic  IconShape=distinctive  AllPortsSameDT=off  OutDataTypeStr=boolean
  Abs4 : Abs
  Abs5 : Abs  ZeroCross=off
  Abs6 : Abs
  Abs7 : Abs  ZeroCross=off
  Compare To Constant{4..7} (4 alike) : simulink/Logic and Bit Operations/Compare To Constant  relop=<=  const=0.5  OutDataTypeStr=boolean
  Demux1 : Demux  Outputs=2
  Transport Delay2 : TransportDelay
  Transport Delay3 : TransportDelay
  Out1 : Outport  OutputWhenDisabled=reset  InitialOutput=0
  wires:
  AND4/1 -> AND6/2
  Abs4/1 -> Compare To Constant4/1
  AND3/1 -> AND6/1
  Abs5/1 -> Compare To Constant5/1
  Transport Delay2/1 -> Abs4/1
  Compare To Constant5/1 -> AND3/1
  Abs6/1 -> Compare To Constant6/1
  AND6/1 -> Out1/1
  Demux1/2 -> Transport Delay3/1, Abs7/1
  virtual errors/1 -> Demux1/1
  Compare To Constant7/1 -> AND4/1
  Compare To Constant4/1 -> AND3/2
  Compare To Constant6/1 -> AND4/2
  Demux1/1 -> Abs5/1, Transport Delay2/1
  Transport Delay3/1 -> Abs6/1
  Abs7/1 -> Compare To Constant7/1

== system gap_generation_platoon/p3/ACC/Headway error ==
  xf : Inport
  vf : Inport  Port=2
  xl : Inport  Port=3
  lcFlag : Inport  Port=4
  Compare To Constant : simulink/Logic and Bit Operations/Compare To Constant  relop=<=  const=0  OutDataTypeStr=boolean
  Demux : Demux  Outputs=2
  Demux1 : Demux  Outputs=2
  Integrator : Integrator  InitialCondition=[h d0]
  Multiply : Product
  Mux : Mux  Inputs=2
  Mux1 : Mux  Inputs=2
  Product : Product
  Sum : Sum  Inputs=-+|
  Sum1 : Sum  Inputs=++|
  Sum2 : Sum  Inputs=+-|
  Sum3 : Sum  Inputs=|++
  Sum4 : Sum  Inputs=|+-
  Sum5 : Sum  Inputs=+-|
  Sum6 : Sum  Inputs=|++
  Switch : Switch  Criteria=u2 > Threshold
  d0 : Constant  Value=d0
  d0Lc : Constant  Value=d0Lc
  h : Constant  Value=h
  hFilterGain : Gain  Gain=hFilterGain
  hLc : Constant  Value=hLc
  vLen : Constant  Value=lr+lf
  eh : Outport
  "gap " : Outport  Port=2
  unsafeFlag : Outport  Port=3
  wires:
  vLen/1 -> Sum1/1
  Multiply/1 -> Sum3/1
  Sum/1 -> Sum5/1, "gap "/1, Sum2/1  "gap"
  xf/1 -> Sum1/2
  Sum3/1 -> Sum2/2  "desired  gap"
  vf/1 -> Product/1, Multiply/1
  Sum1/1 -> Sum/1  "x (front bumber)"
  xl/1 -> Sum/2
  h/1 -> Mux/1
  Switch/1 -> Sum4/1
  Sum4/1 -> hFilterGain/1
  Integrator/1 -> Sum4/2, Demux/1
  lcFlag/1 -> Switch/2
  Sum2/1 -> eh/1
  d0/1 -> Mux/2
  Mux/1 -> Demux1/1, Switch/3  "min safe gap"
  hLc/1 -> Mux1/1
  d0Lc/1 -> Mux1/2
  Mux1/1 -> Switch/1
  Demux/1 -> Multiply/2  "time headway"
  Demux/2 -> Sum3/2  "gap at  standstill"
  hFilterGain/1 -> Integrator/1
  Sum5/1 -> Compare To Constant/1
  Compare To Constant/1 -> unsafeFlag/1
  Demux1/1 -> Product/2  "time headway"
  Product/1 -> Sum6/1
  Demux1/2 -> Sum6/2  "gap at  standstill"
  Sum6/1 -> Sum5/2  "safe  gap"

== system gap_generation_platoon/p3/ACC-v/Headway error ==
  xf : Inport
  vf : Inport  Port=2
  xl : Inport  Port=3
  lcFlag : Inport  Port=4
  Demux : Demux  Outputs=2
  Integrator : Integrator  InitialCondition=h
  Multiply : Product
  Mux : Mux  Inputs=2
  Mux1 : Mux  Inputs=2
  Sum : Sum  Inputs=-+|
  Sum1 : Sum  Inputs=++|
  Sum2 : Sum  Inputs=+-|
  Sum3 : Sum  Inputs=|++
  Sum4 : Sum  Inputs=|+-
  Switch : Switch  Criteria=u2 > Threshold
  d0 : Constant  Value=d0
  d0Lc : Constant  Value=d0Lc
  h : Constant  Value=h
  hFilterGain : Gain  Gain=hFilterGain
  hLc : Constant  Value=hLc
  vLen : Constant  Value=lr+lf
  eh : Outport
  "gap " : Outport  Port=2
  wires:
  vLen/1 -> Sum1/1
  Multiply/1 -> Sum3/1
  Sum/1 -> "gap "/1, Sum2/1  "gap"
  xf/1 -> Sum1/2
  Sum3/1 -> Sum2/2  "desired  gap"
  vf/1 -> Multiply/1
  Sum1/1 -> Sum/1  "x (front bumber)"
  xl/1 -> Sum/2
  h/1 -> Mux/1
  Switch/1 -> Sum4/1
  hFilterGain/1 -> Integrator/1
  Sum4/1 -> hFilterGain/1
  Integrator/1 -> Sum4/2, Demux/1
  lcFlag/1 -> Switch/2
  Sum2/1 -> eh/1
  d0/1 -> Mux/2
  Mux/1 -> Switch/3
  hLc/1 -> Mux1/1
  d0Lc/1 -> Mux1/2
  Mux1/1 -> Switch/1
  Demux/1 -> Multiply/2  "time headway"
  Demux/2 -> Sum3/2  "gap at  standstill"

== system gap_generation_platoon/p3/ACC-v/Triggered Subsystem ==
  Trigger : TriggerPort  VariantControl=Variant
  Constant : Constant
  Out1 : Outport  InitialOutput=0
  wires:
  Constant/1 -> Out1/1

== system gap_generation_platoon/p3/ACC-v/Triggered Subsystem1 ==
  Trigger : TriggerPort  VariantControl=Variant
  Constant : Constant  Value=0
  Out1 : Outport  InitialOutput=1
  wires:
  Constant/1 -> Out1/1

== system gap_generation_platoon/p3/Detect steady state/Subsystem ==
  virtual errors : Inport
  Enable : EnablePort
  AND3 : Logic  IconShape=distinctive  AllPortsSameDT=off  OutDataTypeStr=boolean
  AND4 : Logic  IconShape=distinctive  AllPortsSameDT=off  OutDataTypeStr=boolean
  AND6 : Logic  IconShape=distinctive  AllPortsSameDT=off  OutDataTypeStr=boolean
  Abs4 : Abs
  Abs5 : Abs  ZeroCross=off
  Abs6 : Abs
  Abs7 : Abs  ZeroCross=off
  Compare To Constant{4..7} (4 alike) : simulink/Logic and Bit Operations/Compare To Constant  relop=<=  const=0.5  OutDataTypeStr=boolean
  Demux1 : Demux  Outputs=2
  Transport Delay2 : TransportDelay
  Transport Delay3 : TransportDelay
  Out1 : Outport  OutputWhenDisabled=reset  InitialOutput=0
  wires:
  Abs7/1 -> Compare To Constant7/1
  Transport Delay3/1 -> Abs6/1
  Demux1/1 -> Transport Delay2/1, Abs5/1
  Compare To Constant6/1 -> AND4/2
  Compare To Constant4/1 -> AND3/2
  Compare To Constant7/1 -> AND4/1
  virtual errors/1 -> Demux1/1
  Demux1/2 -> Abs7/1, Transport Delay3/1
  AND6/1 -> Out1/1
  Abs6/1 -> Compare To Constant6/1
  Compare To Constant5/1 -> AND3/1
  Transport Delay2/1 -> Abs4/1
  Abs5/1 -> Compare To Constant5/1
  AND3/1 -> AND6/1
  Abs4/1 -> Compare To Constant4/1
  AND4/1 -> AND6/2
